simulink model "Clarke_Test"  (R2022a)
settings: Solver=VariableStepAuto  StartTime=0.0  StopTime=10.0  RelTol=1e-3
libraries: MyPMSMLibrary x1
settings Model: Creator=jff_1  LastModifiedBy=jff_1

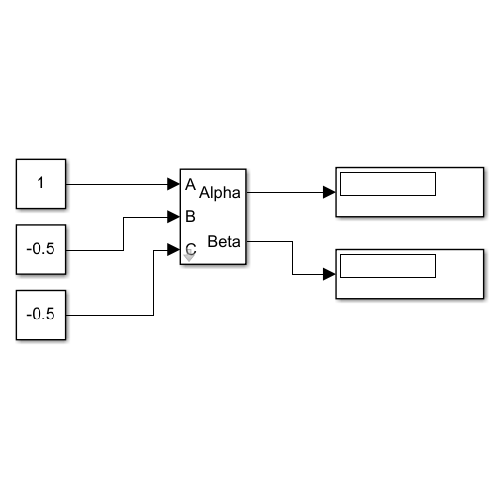
[thumbnail: Simulink's stored preview of the top-level diagram]
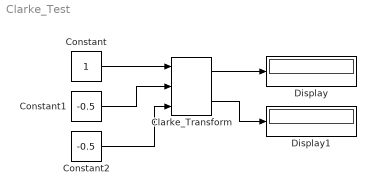
== system Clarke_Test ==
  Clarke_Transform : MyPMSMLibrary/Clarke_Transform
  Constant : Constant
  Constant1 : Constant  Value=-0.5
  Constant2 : Constant  Value=-0.5
  Display : Display
  Display1 : Display
  wires:
  Constant/1 -> Clarke_Transform/1
  Constant1/1 -> Clarke_Transform/2
  Constant2/1 -> Clarke_Transform/3
  Clarke_Transform/1 -> Display/1
  Clarke_Transform/2 -> Display1/1
